simulink model "Robust_design_step_validation"  (R2025b)
settings: Solver=VariableStepAuto  StartTime=0.0  StopTime=20  FixedStep=0.001  RelTol=1e-3
undefined symbols (not defined in the file): daq, degs2rpm, den_G, drv, K, Nu, num_G, Nx, rdp, rpm2rads, sens, Ts, u_bar_max
settings Model: Creator=Enrico  LastModifiedBy=Enrico
settings DataIOCC: ReturnWorkspaceOutputsName=out_black_box

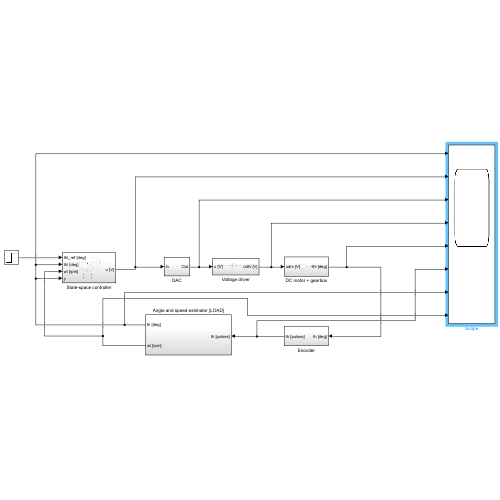
[thumbnail: Simulink's stored preview of the top-level diagram]
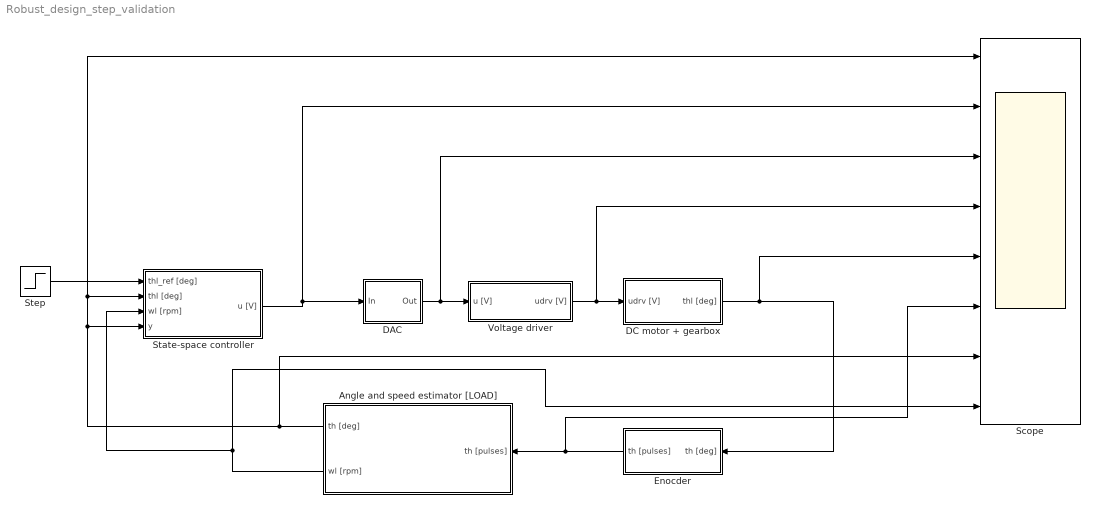
== system Robust_design_step_validation ==
  Angle and speed estimator [LOAD] : Subsystem
  DAC : Subsystem
  DC motor + gearbox : Subsystem
  Enocder : Subsystem
  Scope : Scope  NumInputPorts=8
      settings: ActiveDisplayYMinimum=-5.1559952372592495  ActiveDisplayYMaximum=46.403957135333251
  State-space controller : Subsystem
  Step : Step  After=40  SampleTime=0
  Voltage driver : Subsystem
  wires:
  State-space controller/1(u [V]) -> Scope/2, DAC/1(In)
  DAC/1(Out) -> Scope/3, Voltage driver/1(u [V])
  Step/1 -> State-space controller/1(thl_ref [deg])
  Enocder/1(th [pulses]) -> Scope/6, Angle and speed estimator [LOAD]/1(th [pulses])
  Voltage driver/1(udrv [V]) -> Scope/4, DC motor + gearbox/1(udrv [V])
  DC motor + gearbox/1(thl [deg]) -> Scope/5, Enocder/1(th [deg])
  Angle and speed estimator [LOAD]/1(th [deg]) -> State-space controller/4(y), State-space controller/2(thl [deg]), Scope/1, Scope/7
  Angle and speed estimator [LOAD]/2(wl [rpm]) -> State-space controller/3(wl [rpm]), Scope/8

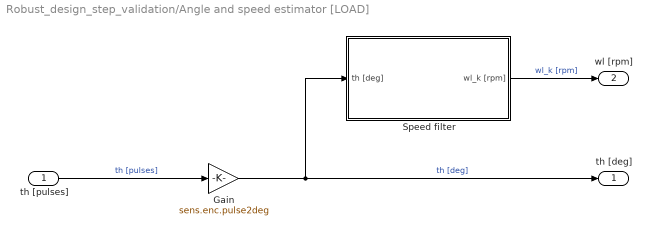
== system Robust_design_step_validation/Angle and speed estimator [LOAD] ==
  th [pulses] : Inport
  Gain : Gain  Gain=sens.enc.pulse2deg
  Speed filter : Subsystem
  th [deg] : Outport
  wl [rpm] : Outport  Port=2
  wires:
  Speed filter/1(wl_k [rpm]) -> wl [rpm]/1  "wl_k [rpm]"
  th [pulses]/1 -> Gain/1  "th [pulses]"
  Gain/1 -> Speed filter/1(th [deg]), th [deg]/1  "th [deg]"

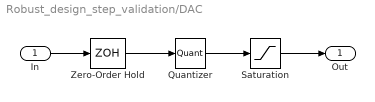
== system Robust_design_step_validation/DAC ==
  In : Inport
  Quantizer : Quantizer  QuantizationInterval=daq.dac.q
  Saturation : Saturate  UpperLimit=daq.dac.fs  LowerLimit=-daq.dac.fs
  Zero-Order Hold : ZeroOrderHold  SampleTime=Ts
  Out : Outport
  wires:
  Quantizer/1 -> Saturation/1
  In/1 -> Zero-Order Hold/1
  Zero-Order Hold/1 -> Quantizer/1
  Saturation/1 -> Out/1

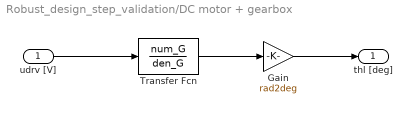
== system Robust_design_step_validation/DC motor + gearbox ==
  udrv [V] : Inport
  Gain : Gain  Gain=rad2deg
  Transfer Fcn : TransferFcn  Numerator=num_G  Denominator=den_G
  thl [deg] : Outport
  wires:
  udrv [V]/1 -> Transfer Fcn/1
  Transfer Fcn/1 -> Gain/1
  Gain/1 -> thl [deg]/1

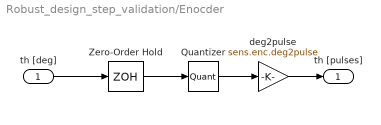
== system Robust_design_step_validation/Enocder ==
  th [deg] : Inport
  Quantizer : Quantizer  QuantizationInterval=sens.enc.pulse2deg
  Zero-Order Hold : ZeroOrderHold  SampleTime=Ts
  deg2pulse : Gain  Gain=sens.enc.deg2pulse
  th [pulses] : Outport
  wires:
  Quantizer/1 -> deg2pulse/1
  th [deg]/1 -> Zero-Order Hold/1
  Zero-Order Hold/1 -> Quantizer/1
  deg2pulse/1 -> th [pulses]/1

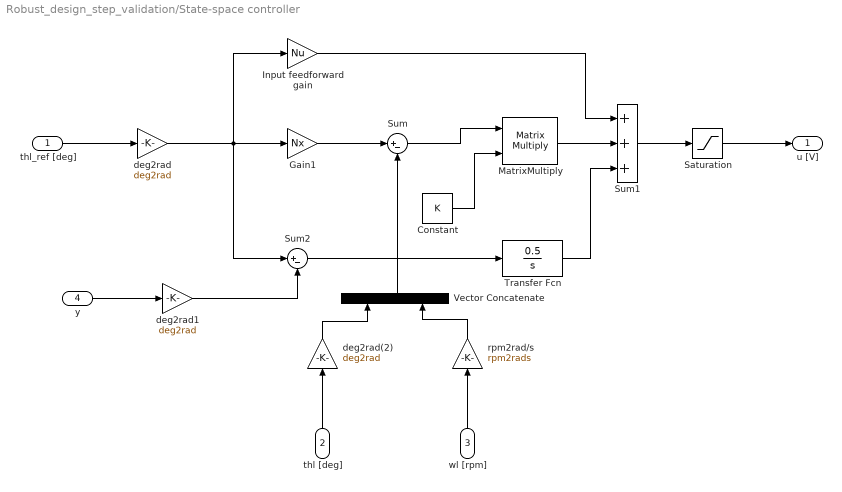
== system Robust_design_step_validation/State-space controller ==
  thl_ref [deg] : Inport
  thl [deg] : Inport  Port=2
  wl [rpm] : Inport  Port=3
  y : Inport  Port=4
  Constant : Constant  Value=K
  Gain1 : Gain  Gain=Nx
  Input feedforward gain : Gain  Gain=Nu
  MatrixMultiply : Product  Multiplication=Matrix(*)
  Saturation : Saturate  UpperLimit=u_bar_max  LowerLimit=-u_bar_max
  Sum : Sum  Inputs=|+-
  Sum1 : Sum  Inputs=+++
  Sum2 : Sum  Inputs=|+-
  Transfer Fcn : TransferFcn  Numerator=[0.5]  Denominator=[1 0]
  Vector Concatenate : Concatenate
  deg2rad : Gain  Gain=deg2rad
  deg2rad(2) : Gain  Gain=deg2rad
  deg2rad1 : Gain  Gain=deg2rad
  rpm2rad/s : Gain  Gain=rpm2rads
  u [V] : Outport
  wires:
  rpm2rad/s/1 -> Vector Concatenate/2
  Gain1/1 -> Sum/1
  Sum1/1 -> Saturation/1
  thl [deg]/1 -> deg2rad(2)/1
  deg2rad/1 -> Sum2/1, Gain1/1, Input feedforward gain/1
  deg2rad(2)/1 -> Vector Concatenate/1
  thl_ref [deg]/1 -> deg2rad/1
  wl [rpm]/1 -> rpm2rad/s/1
  Input feedforward gain/1 -> Sum1/1
  Vector Concatenate/1 -> Sum/2
  Saturation/1 -> u [V]/1
  Sum/1 -> MatrixMultiply/1
  Constant/1 -> MatrixMultiply/2
  MatrixMultiply/1 -> Sum1/2
  Transfer Fcn/1 -> Sum1/3
  Sum2/1 -> Transfer Fcn/1
  y/1 -> deg2rad1/1
  deg2rad1/1 -> Sum2/2

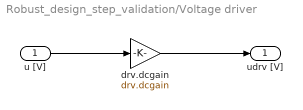
== system Robust_design_step_validation/Voltage driver ==
  u [V] : Inport
  drv.dcgain : Gain  Gain=drv.dcgain
  udrv [V] : Outport
  wires:
  u [V]/1 -> drv.dcgain/1
  drv.dcgain/1 -> udrv [V]/1

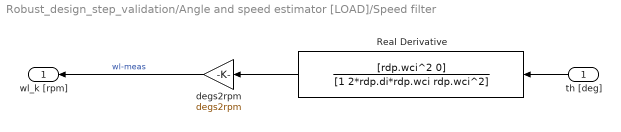
== system Robust_design_step_validation/Angle and speed estimator [LOAD]/Speed filter ==
  th [deg] : Inport
  Real Derivative : TransferFcn  Numerator=[rdp.wci^2 0]  Denominator=[1 2*rdp.di*rdp.wci rdp.wci^2]
  degs2rpm : Gain  Gain=degs2rpm
  wl_k [rpm] : Outport
  wires:
  th [deg]/1 -> Real Derivative/1
  degs2rpm/1 -> wl_k [rpm]/1  "wl-meas"
  Real Derivative/1 -> degs2rpm/1
